simulink model "ac_v_control_mode_1"  (R2021a)
settings: Solver=ode23tb  StartTime=0.0  StopTime=0.1  MaxStep=1e-4  RelTol=1e-3
libraries: spsThyristorLib x6, spsSeriesRLCBranchLib x3, spspowerguiLib x2, spsThreePhaseVIMeasurementLib x1, spsVoltageMeasurementLib x1, spsGroundLib x1, spsThreePhaseProgrammableVoltageSourceLib x1
settings Model: Creator=AHMED  LastModifiedBy=AHMED

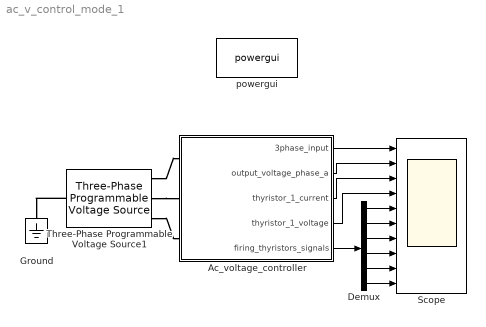
== system ac_v_control_mode_1 ==
  Ac_voltage_controller : Subsystem  mask{angle=30}
      mask prompts: angle "firing_angle"
  Demux : Demux  Outputs=6
  Ground : spsGroundLib/Ground  LConnTagsString=a
  Scope : Scope  NumInputPorts=10
  Three-Phase Programmable Voltage Source1 : spsThreePhaseProgrammableVoltageSourceLib/Three-Phase Programmable Voltage Source  PositiveSequence="[220  0 50]"  VariationEntity=None  VariationType=Table of time-amplitude pairs  VariationTypeAlt=Step  VariationStep=0.5  VariationRate=10  VariationMagnitude=0.3  VariationFrequency=2  VariationTiming=[1 2]  VariationPhaseA=off  Amplitudes=[1 0.8 1.2 1.0]  TimeValues=[0 0.1 0.15 0.2]  HarmonicGeneration=off  HarmonicA=[3 0.2 -25 0]  HarmonicB=[2 0.15 35 2]  Timing="[0.05  3]"  BusType=swing  Pref=0  Qref=0  Qmin=-inf  Qmax=inf
  powergui : spspowerguiLib/powergui  Priority=1  SimulationMode=Continuous  SampleTime=50e-6  frequency=60  Iterations=50  frequencyindice=50  Pbase=100e6  ErrMax=1e-4  UnitsV=kV  UnitsW=MW  buscounter=0  FunctionMessages=off  echomessages=off  EnableUseOfTLC=off  CurrentSourceSwitches=off  DisableSnubberDevices=off  DisableRonSwitches=off  DisableVfSwitches=off  DisplayEquations=off  AutomaticDiscreteSolvers=off  SolverType=Tustin/Backward Euler (TBE)  Interpol=off  ExternalGateDelay=off  methode=off  Ts=100  x0status=blocks  SPID=on  SwTol=0  HookPort=off  NonlinearTolerance=1e-4  nMaxIteration=100  ContinueOnMaxIteration=off  RestoreLinks=warning  ResistiveCurrentMeasurement=off  Frange=[0:2:500]  Ylog=off  Xlog=on  ShowGrid=off  save=off  variable=ZData  structure=0  ZoomFFT=off  StartTime=0.0  cycles=1  DisplayStyle=1  fundamental=60  FreqAxis=off  MaxFrequency=1000  frequencyindicesteady=1  RmsSteady=1  display=off
  wires:
  Ac_voltage_controller/1(3phase_input) -> Scope/1
  Ac_voltage_controller/2(output_voltage_phase_a) -> Scope/2
  Demux/2 -> Scope/6
  Demux/3 -> Scope/7
  Demux/4 -> Scope/8
  Demux/5 -> Scope/9
  Demux/6 -> Scope/10
  Ac_voltage_controller/5(firing_thyristors_signals) -> Demux/1
  Ac_voltage_controller/3(thyristor_1_current) -> Scope/3
  Ac_voltage_controller/4(thyristor_1_voltage) -> Scope/4
  Demux/1 -> Scope/5
  connections:
  Three-Phase Programmable Voltage Source1/RConn1 -- Ac_voltage_controller/LConn1
  Three-Phase Programmable Voltage Source1/RConn2 -- Ac_voltage_controller/LConn2
  Three-Phase Programmable Voltage Source1/RConn3 -- Ac_voltage_controller/LConn3
  Three-Phase Programmable Voltage Source1/LConn1 -- Ground/LConn1

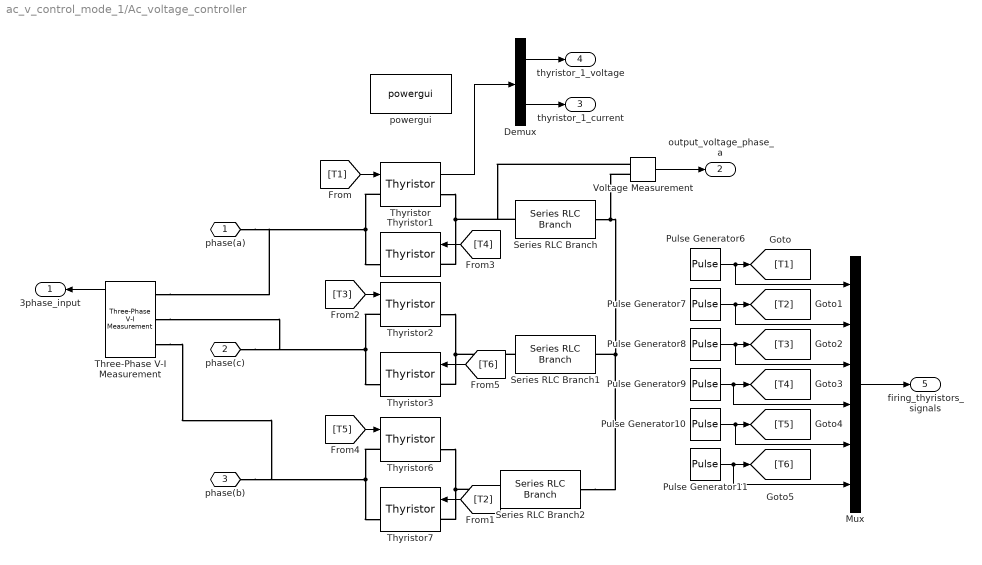
== system ac_v_control_mode_1/Ac_voltage_controller ==
  Demux : Demux  Outputs=2
  Mux : Mux  Inputs=6
  Pulse Generator10 : DiscretePulseGenerator  PulseType=Time based  Period=0.02  PulseWidth=60  PhaseDelay=(0.02/360)*(angle+240)
  Pulse Generator11 : DiscretePulseGenerator  PulseType=Time based  Period=0.02  PulseWidth=60  PhaseDelay=(0.02/360)*(angle+300)
  Pulse Generator6 : DiscretePulseGenerator  PulseType=Time based  Period=0.02  PulseWidth=60  PhaseDelay=(0.02/360)*(angle)
  Pulse Generator7 : DiscretePulseGenerator  PulseType=Time based  Period=0.02  PulseWidth=60  PhaseDelay=(0.02/360)*(angle+60)
  Pulse Generator8 : DiscretePulseGenerator  PulseType=Time based  Period=0.02  PulseWidth=60  PhaseDelay=(0.02/360)*(angle+120)
  Pulse Generator9 : DiscretePulseGenerator  PulseType=Time based  Period=0.02  PulseWidth=60  PhaseDelay=(0.02/360)*(angle+180)
  Series RLC Branch : spsSeriesRLCBranchLib/Series RLC Branch  LConnTagsString=__new0  RConnTagsString=__new0  BranchType=R  Resistance=50  Inductance=1e-3  SetiL0=off  InitialCurrent=0  Capacitance=1e-6  Setx0=off  InitialVoltage=0  Measurements=None
  Series RLC Branch1 : spsSeriesRLCBranchLib/Series RLC Branch  LConnTagsString=__new0  RConnTagsString=__new0  BranchType=R  Resistance=50  Inductance=1e-3  SetiL0=off  InitialCurrent=0  Capacitance=1e-6  Setx0=off  InitialVoltage=0  Measurements=None
  Series RLC Branch2 : spsSeriesRLCBranchLib/Series RLC Branch  LConnTagsString=__new0  RConnTagsString=__new0  BranchType=R  Resistance=50  Inductance=1e-3  SetiL0=off  InitialCurrent=0  Capacitance=1e-6  Setx0=off  InitialVoltage=0  Measurements=None
  Three-Phase V-I Measurement : spsThreePhaseVIMeasurementLib/Three-Phase V-I Measurement  VoltageMeasurement=phase-to-ground  SetLabelV=off  LabelV=Vabc  Vpu=off  VpuLL=off  CurrentMeasurement=yes  SetLabelI=off  LabelI=Iabc  Ipu=off  Pbase=100e6  Vbase=500e3  OutputType=Complex  PhasorSimulation=off  PSBequivalent=0
  Thyristor{,1..3,6..7} (6 alike) : spsThyristorLib/Thyristor  Ron=0.001  Lon=0  Vf=0.8  IC=0  Rs=500  Cs=250e-9  Measurements=on
  Voltage Measurement : spsVoltageMeasurementLib/Voltage Measurement  PhasorSimulation=off  OutputType=Complex  PSBequivalent=0
  powergui : spspowerguiLib/powergui  Priority=1  SimulationMode=Continuous  SampleTime=50e-6  frequency=60  Iterations=50  frequencyindice=50  Pbase=100e6  ErrMax=1e-4  UnitsV=kV  UnitsW=MW  buscounter=0  FunctionMessages=off  echomessages=off  EnableUseOfTLC=off  CurrentSourceSwitches=off  DisableSnubberDevices=off  DisableRonSwitches=off  DisableVfSwitches=off  DisplayEquations=off  AutomaticDiscreteSolvers=off  SolverType=Tustin/Backward Euler (TBE)  Interpol=off  ExternalGateDelay=off  methode=off  Ts=100  x0status=blocks  SPID=on  SwTol=0  HookPort=off  NonlinearTolerance=1e-4  nMaxIteration=100  ContinueOnMaxIteration=off  RestoreLinks=warning  ResistiveCurrentMeasurement=off  Frange=[0:2:500]  Ylog=off  Xlog=on  ShowGrid=off  save=off  variable=ZData  structure=0  ZoomFFT=off  StartTime=0.0  cycles=1  DisplayStyle=1  fundamental=60  FreqAxis=off  MaxFrequency=1000  frequencyindicesteady=1  RmsSteady=1  display=off
  phase(a) : PMIOPort  Side=Left
  phase(c) : PMIOPort  Port=2  Side=Left
  phase(b) : PMIOPort  Port=3  Side=Left
  3phase_input : Outport
  output_voltage_phase_a : Outport  Port=2
  thyristor_1_current : Outport  Port=3
  thyristor_1_voltage : Outport  Port=4
  firing_thyristors_signals : Outport  Port=5
  wires:
  Pulse Generator8/1 -> Mux/3, [T3]
  Pulse Generator7/1 -> Mux/2, [T2]
  Pulse Generator6/1 -> Mux/1, [T1]
  [T3] -> Thyristor2/1
  [T1] -> Thyristor/1
  Pulse Generator9/1 -> Mux/4, [T4]
  Voltage Measurement/1 -> output_voltage_phase_a/1
  [T6] -> Thyristor3/1
  Pulse Generator11/1 -> Mux/6, [T6]
  [T5] -> Thyristor6/1
  [T2] -> Thyristor7/1
  Pulse Generator10/1 -> Mux/5, [T5]
  [T4] -> Thyristor1/1
  Three-Phase V-I Measurement/1 -> 3phase_input/1
  Mux/1 -> firing_thyristors_signals/1
  Demux/1 -> thyristor_1_voltage/1
  Demux/2 -> thyristor_1_current/1
  Thyristor/1 -> Demux/1
  connections:
  Thyristor2/RConn1 -- Series RLC Branch1/LConn1 -- Thyristor3/LConn1
  Series RLC Branch/RConn1 -- Voltage Measurement/LConn2 -- Series RLC Branch2/RConn1 -- Series RLC Branch1/RConn1
  Thyristor6/RConn1 -- Series RLC Branch2/LConn1 -- Thyristor7/LConn1
  Thyristor2/LConn1 -- Three-Phase V-I Measurement/LConn2 -- phase(c)/RConn1 -- Thyristor3/RConn1
  Thyristor/LConn1 -- Three-Phase V-I Measurement/LConn1 -- phase(a)/RConn1 -- Thyristor1/RConn1
  Thyristor/RConn1 -- Voltage Measurement/LConn1 -- Series RLC Branch/LConn1 -- Thyristor1/LConn1
  Thyristor6/LConn1 -- Three-Phase V-I Measurement/LConn3 -- phase(b)/RConn1 -- Thyristor7/RConn1
